simulink model "forceGloveCalibration"  (R2017a)
settings: Solver=ode5  StartTime=0.0  StopTime=10  FixedStep=Ts_sim  RelTol=1e-3  EnableMultiTasking=on
libraries: robotlib x1
settings Model: Creator=Clark  LastModifiedBy=jacob
settings DataIOCC: LimitDataPoints=on  SaveFormat=Array
settings OptimizationCC: LifeSpan=inf
settings DebuggingCC: SFUnexpectedBacktrackingDiag=warning  SFNoUnconditionalDefaultTransitionDiag=warning  SFExecutionAtInitializationDiag=none
settings HardwareCC: ProdBitPerPointer=32  ProdBitPerSizeT=32  ProdBitPerPtrDiffT=32  ProdLargestAtomicFloat=None  ProdIntDivRoundTo=Undefined  ProdEndianess=Unspecified  ProdWordSize=32  ProdHWDeviceType=32-bit Generic
settings ModelReferenceCC: PropagateSignalLabelsOutOfModel=off
settings GRTTargetCC: TargetLangStandard=C89/C90 (ANSI)  GeneratePreprocessorConditionals=Disable all
settings ConfigComp: CovMetricSettings=dw  CovHtmlReporting=on  CovSaveCumulativeToWorkspaceVar=on  CovSaveSingleToWorkspaceVar=on  CovExternalEMLEnable=off

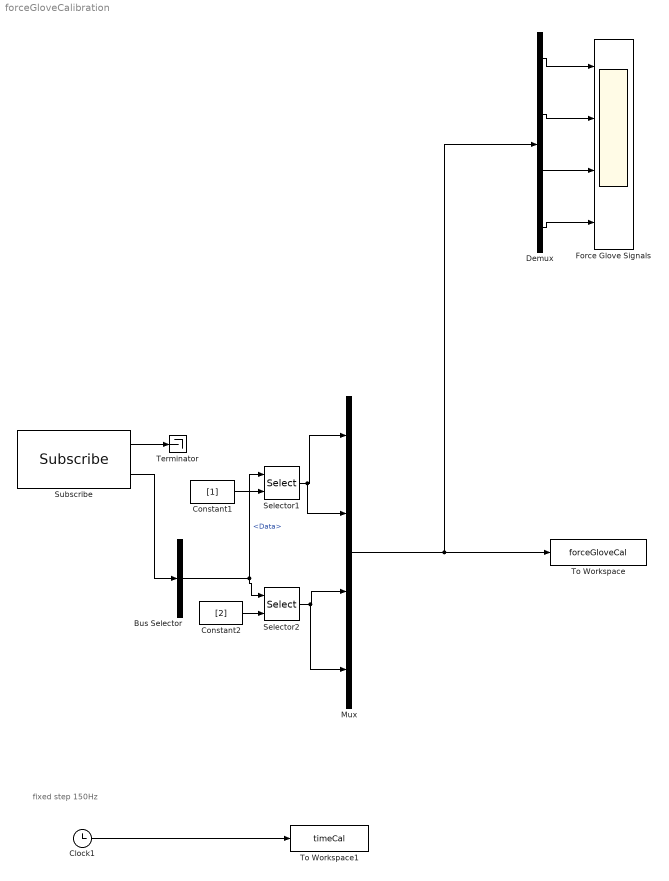
== system forceGloveCalibration ==
  note: fixed step 150Hz
  Bus Selector : BusSelector  OutputSignals=Data
  Clock1 : Clock
  Constant1 : Constant  Value=[1]
  Constant2 : Constant  Value=[2]
  Demux : Demux
  Force Glove Signals : Scope  NumInputPorts=4
  Mux : Mux
  Selector1 : Selector  IndexOptions=Index vector (port)  Indices=[1 3]  OutputSizes=1
  Selector2 : Selector  IndexOptions=Index vector (port)  Indices=[1 3]  OutputSizes=1
  Subscribe : robotlib/Subscribe  SourceLibraryInfo=This block requires Robotics System Toolbox  topicSource=Select from ROS network  topic=/forceGlovePub  messageType=std_msgs/Int16MultiArray  sampleTime=-1  messageQueueLength=1
      settings: SourceProductBaseCode=RO
  Terminator : Terminator
  To Workspace : ToWorkspace  VariableName=forceGloveCal  SampleTime=-1
  To Workspace1 : ToWorkspace  VariableName=timeCal  SampleTime=-1
  wires:
  Demux/1 -> Force Glove Signals/1
  Demux/2 -> Force Glove Signals/2
  Demux/3 -> Force Glove Signals/3
  Demux/4 -> Force Glove Signals/4
  Clock1/1 -> To Workspace1/1
  Constant2/1 -> Selector2/2
  Subscribe/1 -> Terminator/1
  Constant1/1 -> Selector1/2
  Bus Selector/1 -> Selector2/1, Selector1/1  "<Data>"
  Selector2/1 -> Mux/4, Mux/3
  Subscribe/2 -> Bus Selector/1
  Selector1/1 -> Mux/2, Mux/1
  Mux/1 -> To Workspace/1, Demux/1
